simulink model "Prefeeded_Feedback_Control"  (R2025a)
settings: Solver=VariableStepAuto  StartTime=0.0  StopTime=100  RelTol=1e-3
undefined symbols (not defined in the file or in its folder): B, J, K, Kd, Ki, Kp
settings Model: Creator=yurru  LastModifiedBy=yurru

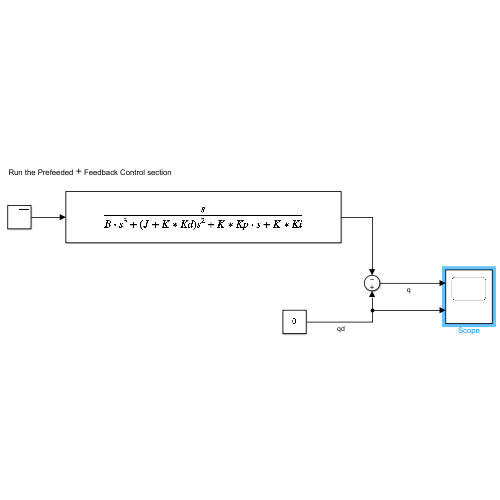
[thumbnail: Simulink's stored preview of the top-level diagram]
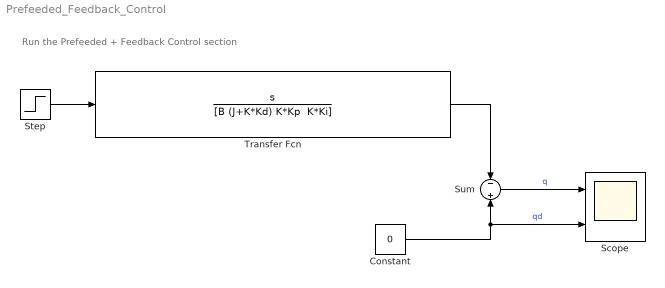
== system Prefeeded_Feedback_Control ==
  note: Run the Prefeeded + Feedback Control section
  Constant : Constant  Value=0
  Scope : Scope  NumInputPorts=2
      settings: ActiveDisplayYMinimum=-0.17322668113417666  ActiveDisplayYMaximum=0.019247409014908543
  Step : Step  SampleTime=0
  Sum : Sum  Inputs=-||+
  Transfer Fcn : TransferFcn  Numerator=[1 0]  Denominator="[B (J+K*Kd) K*Kp  K*Ki]"
  wires:
  Constant/1 -> Sum/2, Scope/2  "qd"
  Sum/1 -> Scope/1  "q"
  Step/1 -> Transfer Fcn/1
  Transfer Fcn/1 -> Sum/1
